simulink model "simulation"  (R2016a)
settings: Solver=VariableStepAuto  SolverMode=SingleTasking  StartTime=0.0  StopTime=27  RelTol=1e-3
settings Model: Creator=Lenovo  LastModifiedBy=Lenovo
settings DataIOCC: ReturnWorkspaceOutputs=on
settings DebuggingCC: SFUnexpectedBacktrackingDiag=error  SFNoUnconditionalDefaultTransitionDiag=error
settings SFSimCC: SimUseLocalCustomCode=on
settings RTWCC: RTWUseLocalCustomCode=on
settings GRTTargetCC: TargetLangStandard=C99 (ISO)
settings ConfigComp: CovMetricSettings=dwe  CovHtmlReporting=off  CovSaveCumulativeToWorkspaceVar=off  CovSaveSingleToWorkspaceVar=off  CovExternalEMLEnable=on

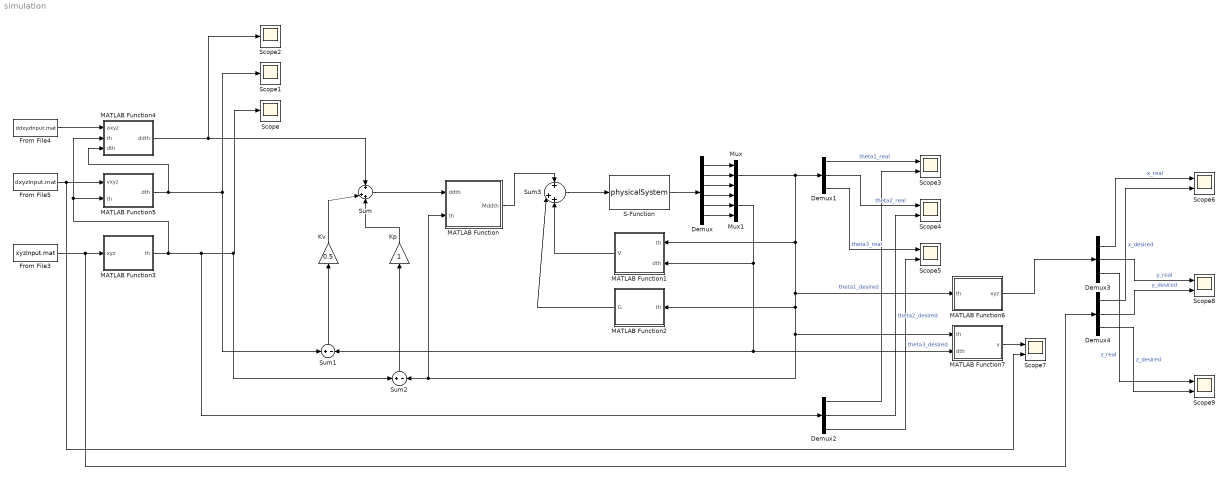
== system simulation ==
  Demux : Demux  Outputs=6
  Demux{1..4} (4 alike) : Demux  Outputs=3
  From File3 : FromFile  FileName=xyzInput.mat
  From File4 : FromFile  FileName=ddxyzInput.mat
  From File5 : FromFile  FileName=dxyzInput.mat
  Kp : Gain
  Kv : Gain  Gain=0.5
  MATLAB Function : MATLAB Function  TreatAsAtomicUnit=on
  MATLAB Function1 : MATLAB Function  TreatAsAtomicUnit=on
  MATLAB Function2 : MATLAB Function  TreatAsAtomicUnit=on
  MATLAB Function3 : MATLAB Function  TreatAsAtomicUnit=on
  MATLAB Function4 : MATLAB Function  TreatAsAtomicUnit=on
  MATLAB Function5 : MATLAB Function  TreatAsAtomicUnit=on
  MATLAB Function6 : MATLAB Function  TreatAsAtomicUnit=on
  MATLAB Function7 : MATLAB Function  TreatAsAtomicUnit=on
  Mux : Mux  Inputs=3
  Mux1 : Mux  Inputs=3
  S-Function : S-Function  FunctionName=physicalSystem  SFunctionDeploymentMode=off  EnableBusSupport=off
  Scope : Scope
  Scope1 : Scope
  Scope2 : Scope
  Scope{3..9} (7 alike) : Scope  NumInputPorts=2
  Sum : Sum  Inputs=+|++
  Sum1 : Sum  Inputs=+|-
  Sum2 : Sum  Inputs=+|-
  Sum3 : Sum  Inputs=+|++
  wires:
  MATLAB Function4/1(ddth) -> Sum/1, Scope2/1
  MATLAB Function5/1(dth) -> MATLAB Function4/3(dth), Scope1/1, Sum1/1
  MATLAB Function3/1(th) -> Demux2/1, Sum2/1, Scope/1, MATLAB Function5/2(th), MATLAB Function4/2(th)
  Kv/1 -> Sum/2
  Kp/1 -> Sum/3
  Sum1/1 -> Kv/1
  Sum2/1 -> Kp/1
  MATLAB Function/1(Mddth) -> Sum3/1
  Sum3/1 -> S-Function/1
  MATLAB Function1/1(V) -> Sum3/3
  MATLAB Function2/1(G) -> Sum3/2
  S-Function/1 -> Demux/1
  Sum/1 -> MATLAB Function/1(ddth)
  Demux/1 -> Mux/1
  Demux/2 -> Mux/2
  Demux/3 -> Mux/3
  Demux/4 -> Mux1/1
  Demux/5 -> Mux1/2
  Demux/6 -> Mux1/3
  Mux/1 -> Demux1/1, MATLAB Function1/1(th), MATLAB Function6/1(th), MATLAB Function2/1(th), MATLAB Function7/1(th), MATLAB Function/2(th), Sum2/2
  Mux1/1 -> MATLAB Function1/2(dth), MATLAB Function7/2(dth), Sum1/2
  Demux1/1 -> Scope3/1  "theta1_real"
  Demux1/2 -> Scope4/1  "theta2_real"
  Demux1/3 -> Scope5/1  "theta3_real"
  Demux2/3 -> Scope5/2  "theta3_desired"
  Demux2/2 -> Scope4/2  "theta2_desired"
  Demux2/1 -> Scope3/2  "theta1_desired"
  From File3/1 -> Demux4/1, MATLAB Function3/1(xyz)
  From File4/1 -> MATLAB Function4/1(axyz)
  From File5/1 -> Scope7/2, MATLAB Function5/1(vxyz)
  MATLAB Function7/1(v) -> Scope7/1
  MATLAB Function6/1(xyz) -> Demux3/1
  Demux3/1 -> Scope6/1  "x_real"
  Demux4/1 -> Scope6/2  "x_desired"
  Demux3/2 -> Scope8/1  "y_real"
  Demux4/2 -> Scope8/2  "y_desired"
  Demux3/3 -> Scope9/1  "z_real"
  Demux4/3 -> Scope9/2  "z_desired"

== matlab function simulation/MATLAB Function1 ==
  data: th input; V output; dth input
function V = funcV(th, dth)
    th2 = th(2);
    th3 = th(3);
    dth1 = dth(1);
    dth2 = dth(2);
    dth3 = dth(3);
    l2 = 135/100;   % [m]
    l3 = 147/100;   % [m]
    m1 = 1.5;       % [kg]
    m2 = 1;         % [kg]
    m3 = 1;         % [kg]
    r = 75/100;    % [m]
    g = 9.8;


V = [dth1.*(dth2.*l2.^2.*m2.*sin(th2.*2.0)+dth2.*l2.^2.*m3.*sin(th2.*2.0).*2.0+dth2.*l3.^2.*m3.*sin(th2.*2.0+th3.*2.0).*4.0+dth3.*l3.^2.*m3.*sin(th2.*2.0+th3.*2.0).*4.0+dth2.*l2.*l3.*m3.*sin(th2.*2.0+th3).*4.0+dth3.*l2.*l3.*m3.*sin(th2.*2.0+th3).*2.0+dth3.*l2.*l3.*m3.*sin(th3).*2.0).*(-1.0./2.0);...
    (l2.*m2.*cos(th2))./2.0+l2.*m3.*cos(th2)+l3.*m3.*cos(th2+th3)-g.*l3.*m3.*cos(th2+th3)-(g.*l2.*m2.*cos(th2))./2.0-g.*l2.*m3.*cos(th2)+(dth1.^2.*l2.^2.*m2.*sin(th2.*2.0))./4.0+(dth1.^2.*l2.^2.*m3.*sin(th2.*2.0))./2.0+dth1.^2.*l3.^2.*m3.*sin(th2.*2.0+th3.*2.0)-dth3.^2.*l2.*l3.*m3.*sin(th3)+dth1.^2.*l2.*l3.*m3.*sin(th2.*2.0+th3)-dth2.*dth3.*l2.*l3.*m3.*sin(th3).*2.0;...
    (l3.*m3.*(cos(th2+th3).*2.0-g.*cos(th2+th3).*2.0+dth1.^2.*l3.*sin(th2.*2.0+th3.*2.0).*2.0+dth1.^2.*l2.*sin(th3)+dth2.^2.*l2.*sin(th3).*2.0+dth1.^2.*l2.*sin(th2.*2.0+th3)))./2.0];

end

== matlab function simulation/MATLAB Function ==
  data: Mddth output; ddth input; th input
function Mddth = funcM(ddth, th)
    th2 = th(2);
    th3 = th(3);
    l2 = 135/100;   % [m]
    l3 = 147/100;   % [m]
    m1 = 1.5;       % [kg]
    m2 = 1;         % [kg]
    m3 = 1;         % [kg]
    r = 75/100;    % [m]
    
    M = reshape( ...
        [(l2.^2.*m2)./4.0+(l2.^2.*m3)./2.0+l3.^2.*m3+(m1.*r.^2)./2.0+l3.^2.*m3.*cos(th2.*2.0+th3.*2.0)+(l2.^2.*m2.*cos(th2.*2.0))./4.0+(l2.^2.*m3.*cos(th2.*2.0))./2.0+l2.*l3.*m3.*cos(th3)+l2.*l3.*m3.*cos(th2.*2.0+th3),0.0,0.0, ...
        0.0,    (l2.^2.*m2)./2.0+l2.^2.*m3+l3.^2.*m3.*2.0+l2.*l3.*m3.*cos(th3).*2.0,l3.*m3.*(l3.*2.0+l2.*cos(th3)), ...
        0.0,    l3.*m3.*(l3.*2.0+l2.*cos(th3)),     l3.^2.*m3.*2.0],...
        [3,3]);
    
    Mddth = M*ddth;
end

== matlab function simulation/MATLAB Function2 ==
  data: th input; G output
function G = funcG(th)
    th2 = th(2);
    th3 = th(3);
    l2 = 135/100;   % [m]
    l3 = 147/100;   % [m]
    m1 = 1.5;       % [kg]
    m2 = 1;         % [kg]
    m3 = 1;         % [kg]


G = [0.0;
    l2.*m2.*cos(th2).*(-1.0./2.0)-l2.*m3.*cos(th2)-l3.*m3.*cos(th2+th3);
    -l3.*m3.*cos(th2+th3)];

end

== matlab function simulation/MATLAB Function3 ==
  data: th output; xyz input
function th = invkine(xyz)
    l2 = 135/100;   % [m]
    l3 = 147/100;   % [m]
    dt = 0.01;      % [s] 时间间隔

    x = xyz(1);
    y = xyz(2);
    z = xyz(3);

    ll = sqrt(x^2+y^2+z^2);
    if ll > l2+l3
        error("It has exceed the working space");
    end

    % 根据几何关系，可以首先算出theta3
    c3 = (x*x+y*y+z*z-l2*l2-l3*l3)/(2*l2*l3);
    tt3 = -acos(c3);
    % theta1也很容易确定
    tt1 = atan2(y, x);
    % theta2
    beta = atan2(z, sqrt(x*x+y*y) );
    phi = acos( (x^2+y^2+z^2+l2^2-l3^2) / (2*l2*sqrt(x^2+y^2+z^2)) );
    tt2 = beta + phi;
    th = [tt1; tt2; tt3];
    
end

== matlab function simulation/MATLAB Function4 ==
  data: axyz input; ddth output; th input; dth input
function ddth = invHessian(axyz, th, dth)

l1 = 138/100;   % [m]
l2 = 135/100;   % [m]
l3 = 147/100;   % [m]

th1 = th(1);
th2 = th(2);
th3 = th(3);
dth1 = dth(1);
dth2 = dth(2);
dth3 = dth(3);
omega = [dth1; dth2; dth3];
a = [axyz(1); axyz(2); axyz(3)];

H1 = reshape([-cos(th1).*(l3.*cos(th2+th3)+l2.*cos(th2)),sin(th1).*(l3.*sin(th2+th3)+l2.*sin(th2)),l3.*sin(th2+th3).*sin(th1),sin(th1).*(l3.*sin(th2+th3)+l2.*sin(th2)),-cos(th1).*(l3.*cos(th2+th3)+l2.*cos(th2)),-l3.*cos(th2+th3).*cos(th1),l3.*sin(th2+th3).*sin(th1),-l3.*cos(th2+th3).*cos(th1),-l3.*cos(th2+th3).*cos(th1)],[3,3]);
H2 = reshape([-sin(th1).*(l3.*cos(th2+th3)+l2.*cos(th2)),-cos(th1).*(l3.*sin(th2+th3)+l2.*sin(th2)),-l3.*sin(th2+th3).*cos(th1),-cos(th1).*(l3.*sin(th2+th3)+l2.*sin(th2)),-sin(th1).*(l3.*cos(th2+th3)+l2.*cos(th2)),-l3.*cos(th2+th3).*sin(th1),-l3.*sin(th2+th3).*cos(th1),-l3.*cos(th2+th3).*sin(th1),-l3.*cos(th2+th3).*sin(th1)],[3,3]);
H3 = reshape([0.0,0.0,0.0,0.0,-l3.*sin(th2+th3)-l2.*sin(th2),-l3.*sin(th2+th3),0.0,-l3.*sin(th2+th3),-l3.*sin(th2+th3)],[3,3]);
J = reshape([-sin(th1).*(l3.*cos(th2+th3)+l2.*cos(th2)),cos(th1).*(l3.*cos(th2+th3)+l2.*cos(th2)),0.0,-cos(th1).*(l3.*sin(th2+th3)+l2.*sin(th2)),-sin(th1).*(l3.*sin(th2+th3)+l2.*sin(th2)),l3.*cos(th2+th3)+l2.*cos(th2),-l3.*sin(th2+th3).*cos(th1),-l3.*sin(th2+th3).*sin(th1),l3.*cos(th2+th3)],[3,3]);
Jinv = inv(J);


temp = [
    omega' * H1 * omega
    omega' * H2 * omega
    omega' * H3 * omega
    ];

ddth = Jinv*( a - temp );

== matlab function simulation/MATLAB Function5 ==
  data: vxyz input; dth output; th input
function dth = invJacobi(vxyz, th)
th1 = th(1);
th2 = th(2);
th3 = th(3);

l1 = 138/100;   % [m]
l2 = 135/100;   % [m]
l3 = 147/100;   % [m]
J = reshape([-sin(th1).*(l3.*cos(th2+th3)+l2.*cos(th2)),cos(th1).*(l3.*cos(th2+th3)+l2.*cos(th2)),0.0,-cos(th1).*(l3.*sin(th2+th3)+l2.*sin(th2)),-sin(th1).*(l3.*sin(th2+th3)+l2.*sin(th2)),l3.*cos(th2+th3)+l2.*cos(th2),-l3.*sin(th2+th3).*cos(th1),-l3.*sin(th2+th3).*sin(th1),l3.*cos(th2+th3)],[3,3]);

Jinv = inv(J);

v = [0; 0; 0];
v(1) = vxyz(1);
v(2) = vxyz(2);
v(3) = vxyz(3);

dth = Jinv*v;

== matlab function simulation/MATLAB Function6 ==
  data: th input; xyz output
function xyz = fkine(th)

%     th2 = th(2);
%     th3 = th(3);
l1 = 138/100;   % [m]
l2 = 135/100;   % [m]
l3 = 147/100;   % [m]
%     m1 = 1.5;       % [kg]
%     m2 = 1;         % [kg]
%     m3 = 1;         % [kg]
%     r = 75/100;    % [m]

T1 = Tmat(0, 0, 0, th(1));
T2 = Tmat(pi/2, 0, 0, th(2));
T3 = Tmat(0, l2, 0, th(3));
TH = Tmat(0, l3, 0, 0);

T0H = T1*T2*T3*TH;

xyz = T0H(1:3, 4);

end



function T = Tmat(alp, a, d, th)
    sa = sin(alp);
    ca = cos(alp);
    st = sin(th);
    ct = cos(th);
    T = [ ct    -st    0    a
         st*ca  ct*ca  -sa  -sa*d
         st*sa  ct*sa  ca   ca*d
          0      0     0      1  ];
end

== matlab function simulation/MATLAB Function7 ==
  data: th input; v output; dth input
function v = jacobi(th, dth)
th1 = th(1);
th2 = th(2);
th3 = th(3);
dth1 = dth(1);
dth2 = dth(2);
dth3 = dth(3);
l1 = 138/100;   % [m]
l2 = 135/100;   % [m]
l3 = 147/100;   % [m]
J = reshape([-sin(th1).*(l3.*cos(th2+th3)+l2.*cos(th2)),cos(th1).*(l3.*cos(th2+th3)+l2.*cos(th2)),0.0,-cos(th1).*(l3.*sin(th2+th3)+l2.*sin(th2)),-sin(th1).*(l3.*sin(th2+th3)+l2.*sin(th2)),l3.*cos(th2+th3)+l2.*cos(th2),-l3.*sin(th2+th3).*cos(th1),-l3.*sin(th2+th3).*sin(th1),l3.*cos(th2+th3)],[3,3]);

omega = [dth(1); dth(2); dth(3)];

v = J * omega;
